simulink subsystem "Motor"  (R2023a)
settings: Solver=VariableStepAuto  StartTime=0.0  StopTime=10.0  RelTol=1e-3
model mask{Un=24, R=10, Ni=14400, Ii=60 * 10^(-3), Kn=600, Km=16 * 10^(-3), L=350 * 10^(-6), J_motor=500 * 10^(-9), vis_friction_coef_motor=0.01}
  mask prompts: Un "nominal voltage"; R "Resistance"; Ni "Idling speed"; Ii "Idling current"; Kn "Speed constant (rpm/V)"; Km "Torque constant"; L "Inductivity"; J_motor "Rotor inertia"; vis_friction_coef_motor "Friction coefficient"
settings Model: Creator=User  LastModifiedBy=User

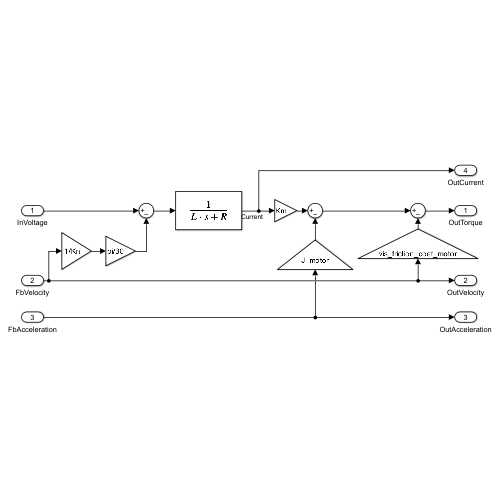
[thumbnail: Simulink's stored preview of the top-level diagram]
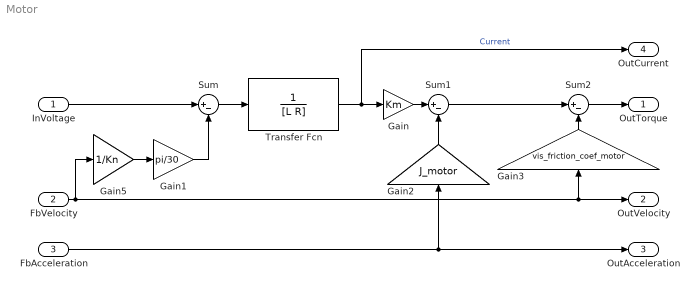
== system Motor ==
  InVoltage : Inport
  FbVelocity : Inport  Port=2
  FbAcceleration : Inport  Port=3
  Gain : Gain  Gain=Km
  Gain1 : Gain  Gain=pi/30
  Gain2 : Gain  Gain=J_motor
  Gain3 : Gain  Gain=vis_friction_coef_motor
  Gain5 : Gain  Gain=1/Kn
  Sum : Sum  Inputs=|+-
  Sum1 : Sum  Inputs=|+-
  Sum2 : Sum  Inputs=|+-
  Transfer Fcn : TransferFcn  Denominator=[L R]
  OutTorque : Outport
  OutVelocity : Outport  Port=2
  OutAcceleration : Outport  Port=3
  OutCurrent : Outport  Port=4
  wires:
  FbVelocity/1 -> OutVelocity/1, Gain3/1, Gain5/1
  Sum1/1 -> Sum2/1
  FbAcceleration/1 -> OutAcceleration/1, Gain2/1
  Sum2/1 -> OutTorque/1
  Sum/1 -> Transfer Fcn/1
  Gain2/1 -> Sum1/2
  Gain3/1 -> Sum2/2
  Gain/1 -> Sum1/1
  Transfer Fcn/1 -> OutCurrent/1, Gain/1  "Current"
  InVoltage/1 -> Sum/1
  Gain5/1 -> Gain1/1
  Gain1/1 -> Sum/2
